simulink model "simulator_P2_2"  (R2021b)
settings: Solver=ode45  StartTime=0.0  StopTime=600  FixedStep=Ts  RelTol=1e-3  EnableMultiTasking=on
values from neighbouring files (symbols this model uses):
  A = [-0.0265 0 0.0884 0;0 -0.0265 0 0.0884; 0 0 -0.0884 0; 0 0 0 -0.0884]    [four_tanks_session2_Michal_Szabo_Michael_Brian_Damkoehler.m]
  A1 = 28    [four_tanks_session2_Michal_Szabo_Michael_Brian_Damkoehler.m]
  a1 = 0.071    [four_tanks_session2_Michal_Szabo_Michael_Brian_Damkoehler.m]
  A2 = 28    [four_tanks_session2_Michal_Szabo_Michael_Brian_Damkoehler.m]
  a2 = 0.071    [four_tanks_session2_Michal_Szabo_Michael_Brian_Damkoehler.m]
  a3 = 0.071    [four_tanks_session2_Michal_Szabo_Michael_Brian_Damkoehler.m]
  A3 = 28    [four_tanks_session2_Michal_Szabo_Michael_Brian_Damkoehler.m]
  a4 = 0.071    [four_tanks_session2_Michal_Szabo_Michael_Brian_Damkoehler.m]
  A4 = 28    [four_tanks_session2_Michal_Szabo_Michael_Brian_Damkoehler.m]
  B = [0.0833 0;0 0.0833; 0 0.0357;0.0357 0]    [four_tanks_session2_Michal_Szabo_Michael_Brian_Damkoehler.m]
  C = [1 0 0 0;0 1 0 0;0 0 1 0;0 0 0 1]    [four_tanks_session2_Michal_Szabo_Michael_Brian_Damkoehler.m]
  D = [0 0;0 0;0 0;0 0]    [four_tanks_session2_Michal_Szabo_Michael_Brian_Damkoehler.m]
  de = 0.025    [four_tanks_session2_Michal_Szabo_Michael_Brian_Damkoehler.m]
  g = 981    [four_tanks_session2_Michal_Szabo_Michael_Brian_Damkoehler.m]
  gamma1 = 0.7    [four_tanks_session2_Michal_Szabo_Michael_Brian_Damkoehler.m]
  gamma2 = 0.7    [four_tanks_session2_Michal_Szabo_Michael_Brian_Damkoehler.m]
  h10 = 4.4847    [four_tanks_session2_Michal_Szabo_Michael_Brian_Damkoehler.m]
  h20 = 4.4847    [four_tanks_session2_Michal_Szabo_Michael_Brian_Damkoehler.m]
  h30 = 0.4036    [four_tanks_session2_Michal_Szabo_Michael_Brian_Damkoehler.m]
  h40 = 0.4036    [four_tanks_session2_Michal_Szabo_Michael_Brian_Damkoehler.m]
  k1 = 3.33    [four_tanks_session2_Michal_Szabo_Michael_Brian_Damkoehler.m]
  k2 = 3.33    [four_tanks_session2_Michal_Szabo_Michael_Brian_Damkoehler.m]
  seed = [1 253 529 751]    [four_tanks_session2_Michal_Szabo_Michael_Brian_Damkoehler.m]
  Ts = 1    [four_tanks_session2_Michal_Szabo_Michael_Brian_Damkoehler.m]
  v10 = 2    [four_tanks_session2_Michal_Szabo_Michael_Brian_Damkoehler.m]
  v20 = 2    [four_tanks_session2_Michal_Szabo_Michael_Brian_Damkoehler.m]
settings Model: Creator=as  LastModifiedBy=szmis
settings SolverCC: AlgebraicLoopSolver=TrustRegion
settings DataIOCC: LimitDataPoints=on  SaveFormat=Array  SignalLoggingSaveFormat=ModelDataLogs  ReturnWorkspaceOutputs=off
settings OptimizationCC: LifeSpan=inf
settings DebuggingCC: SaveWithParameterizedLinksMsg=none  UnderspecifiedInitializationDetection=Classic  MergeDetectMultiDrivingBlocksExec=none  SolverPrmCheckMsg=warning  FcnCallInpInsideContextMsg=warning  SFUnexpectedBacktrackingDiag=warning  SFNoUnconditionalDefaultTransitionDiag=warning  SFExecutionAtInitializationDiag=none  SFMachineParentedDataDiag=warning  ArithmeticOperatorsInVariantConditions=warning
settings HardwareCC: ProdBitPerPointer=32  ProdBitPerSizeT=32  ProdBitPerPtrDiffT=32  ProdLargestAtomicFloat=None  ProdIntDivRoundTo=Undefined  ProdEndianess=Unspecified  ProdWordSize=32  ProdHWDeviceType=32-bit Generic
settings ModelReferenceCC: PropagateSignalLabelsOutOfModel=off
settings SFSimCC: SimUseLocalCustomCode=off  CustomCodeUndefinedFunction=UseInterfaceOnly
settings RTWCC: RTWUseLocalCustomCode=off
settings CodeAppCC: StateflowObjectComments=on
settings GRTTargetCC: TargetLangStandard=C89/C90 (ANSI)  CombineOutputUpdateFcns=off  GRTInterface=on
settings ConfigComp: CovMetricSettings=dw  CovSaveCumulativeToWorkspaceVar=on  CovSaveSingleToWorkspaceVar=on  CovExternalEMLEnable=off

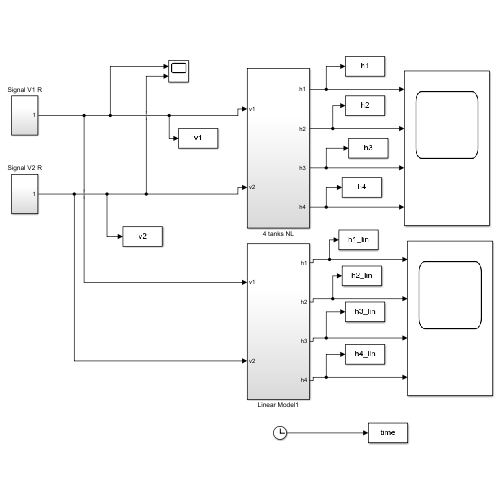
[thumbnail: Simulink's stored preview of the top-level diagram]
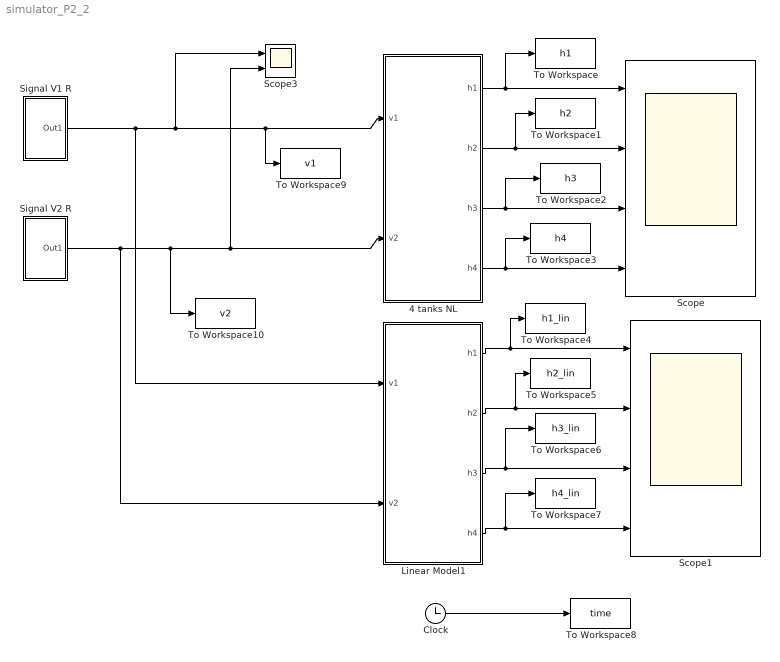
== system simulator_P2_2 ==
  4 tanks NL : Subsystem
  Clock : Clock
  Linear Model1 : Subsystem
  Scope : Scope  NumInputPorts=4
  Scope1 : Scope  NumInputPorts=4
  Scope3 : Scope  NumInputPorts=2
  Signal V1 R : Subsystem
  Signal V2 R : Subsystem
  To Workspace : ToWorkspace  VariableName=h1  SampleTime=Ts
  To Workspace1 : ToWorkspace  VariableName=h2  SampleTime=Ts
  To Workspace10 : ToWorkspace  VariableName=v2  SampleTime=Ts
  To Workspace2 : ToWorkspace  VariableName=h3  SampleTime=Ts
  To Workspace3 : ToWorkspace  VariableName=h4  SampleTime=Ts
  To Workspace4 : ToWorkspace  VariableName=h1_lin  SampleTime=Ts
  To Workspace5 : ToWorkspace  VariableName=h2_lin  SampleTime=Ts
  To Workspace6 : ToWorkspace  VariableName=h3_lin  SampleTime=Ts
  To Workspace7 : ToWorkspace  VariableName=h4_lin  SampleTime=Ts
  To Workspace8 : ToWorkspace  VariableName=time  SampleTime=Ts
  To Workspace9 : ToWorkspace  VariableName=v1  SampleTime=Ts
  wires:
  Signal V1 R/1(Out1) -> Scope3/1, 4 tanks NL/1(v1), To Workspace9/1, Linear Model1/1(v1)
  4 tanks NL/1("h1 ") -> Scope/1, To Workspace/1
  4 tanks NL/2("h2 ") -> Scope/2, To Workspace1/1
  4 tanks NL/3("h3 ") -> Scope/3, To Workspace2/1
  4 tanks NL/4("h4 ") -> Scope/4, To Workspace3/1
  Linear Model1/1(h1) -> Scope1/1, To Workspace4/1
  Linear Model1/2(h2) -> Scope1/2, To Workspace5/1
  Linear Model1/3(h3) -> Scope1/3, To Workspace6/1
  Linear Model1/4(h4) -> Scope1/4, To Workspace7/1
  Clock/1 -> To Workspace8/1
  Signal V2 R/1(Out1) -> 4 tanks NL/2(v2), Scope3/2, To Workspace10/1, Linear Model1/2(v2)

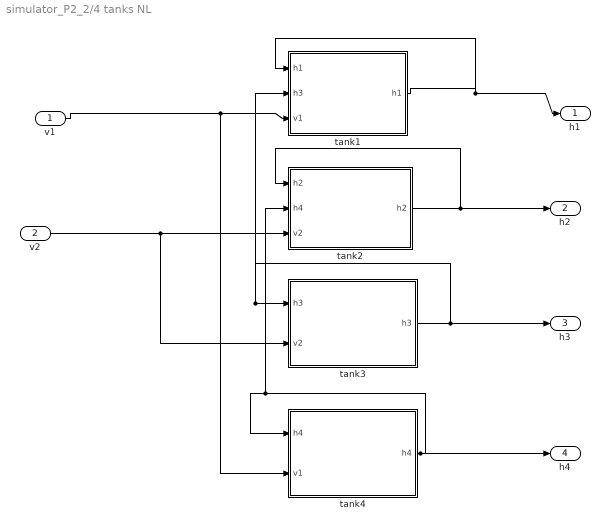
== system simulator_P2_2/4 tanks NL ==
  v1 : Inport
  v2 : Inport  Port=2
  tank1 : Subsystem
  tank2 : Subsystem
  tank3 : Subsystem
  tank4 : Subsystem
  "h1 " : Outport
  "h2 " : Outport  Port=2
  "h3 " : Outport  Port=3
  "h4 " : Outport  Port=4
  wires:
  tank4/1("h4 ") -> tank4/1(h4), tank2/2(h4), "h4 "/1
  tank3/1("h3 ") -> tank3/1(h3), tank1/2(h3), "h3 "/1
  v2/1 -> tank2/3(v2), tank3/2(v2)
  tank2/1("h2 ") -> tank2/1(h2), "h2 "/1
  v1/1 -> tank1/3(v1), tank4/2(v1)
  tank1/1("h1 ") -> tank1/1(h1), "h1 "/1

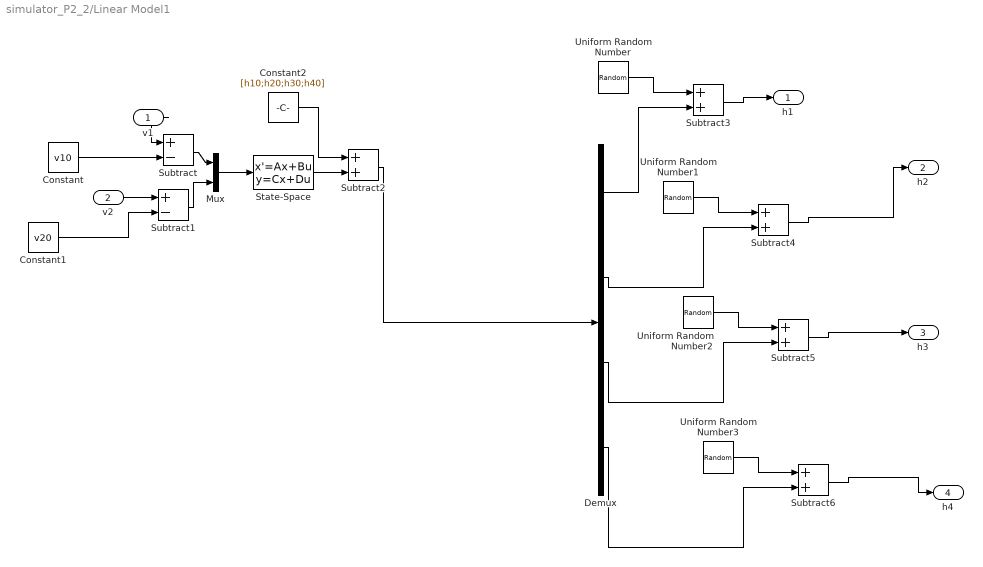
== system simulator_P2_2/Linear Model1 ==
  v1 : Inport
  v2 : Inport  Port=2
  Constant : Constant  Value=v10
  Constant1 : Constant  Value=v20
  Constant2 : Constant  Value=[h10;h20;h30;h40]
  Demux : Demux
  Mux : Mux  Inputs=2
  State-Space : StateSpace  A=A  B=B  C=C  D=D  InitialCondition=0
  Subtract : Sum  Inputs=+-
  Subtract1 : Sum  Inputs=+-
  Subtract{2..6} (5 alike) : Sum
  Uniform Random Number : UniformRandomNumber  Minimum=-de  Maximum=de  Seed=seed(1)  SampleTime=Ts
  Uniform Random Number1 : UniformRandomNumber  Minimum=-de  Maximum=de  Seed=seed(2)  SampleTime=Ts
  Uniform Random Number2 : UniformRandomNumber  Minimum=-de  Maximum=de  Seed=seed(3)  SampleTime=Ts
  Uniform Random Number3 : UniformRandomNumber  Minimum=-de  Maximum=de  Seed=seed(4)  SampleTime=Ts
  h1 : Outport
  h2 : Outport  Port=2
  h3 : Outport  Port=3
  h4 : Outport  Port=4
  wires:
  Mux/1 -> State-Space/1
  Constant/1 -> Subtract/2
  Subtract/1 -> Mux/1
  Subtract1/1 -> Mux/2
  Constant1/1 -> Subtract1/2
  Subtract2/1 -> Demux/1
  Constant2/1 -> Subtract2/1
  State-Space/1 -> Subtract2/2
  v1/1 -> Subtract/1
  v2/1 -> Subtract1/1
  Demux/1 -> Subtract3/2
  Subtract3/1 -> h1/1
  Uniform Random Number/1 -> Subtract3/1
  Demux/2 -> Subtract4/2
  Subtract4/1 -> h2/1
  Uniform Random Number1/1 -> Subtract4/1
  Demux/3 -> Subtract5/2
  Subtract5/1 -> h3/1
  Uniform Random Number2/1 -> Subtract5/1
  Demux/4 -> Subtract6/2
  Subtract6/1 -> h4/1
  Uniform Random Number3/1 -> Subtract6/1

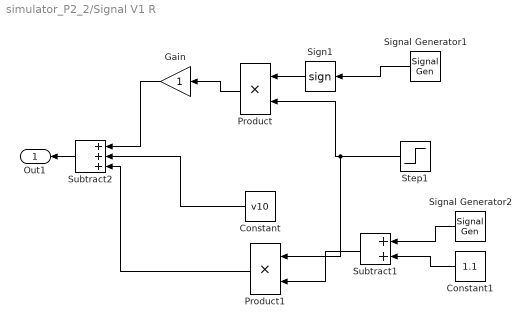
== system simulator_P2_2/Signal V1 R ==
  Constant : Constant  Value=v10
  Constant1 : Constant  Value=1.1
  Gain : Gain
  Product : Product  RndMeth=Zero
  Product1 : Product  RndMeth=Zero
  Sign1 : Signum
  Signal Generator1 : SignalGenerator  WaveForm=random  Amplitude=1.8  Frequency=200
  Signal Generator2 : SignalGenerator  WaveForm=sawtooth  Amplitude=1.1  Frequency=0.005
  Step1 : Step  Time=10  SampleTime=0
  Subtract1 : Sum
  Subtract2 : Sum  Inputs=+++
  Out1 : Outport
  wires:
  Sign1/1 -> Product/1
  Step1/1 -> Product/2, Product1/1
  Constant/1 -> Subtract2/2
  Subtract2/1 -> Out1/1
  Product/1 -> Gain/1
  Gain/1 -> Subtract2/1
  Signal Generator1/1 -> Sign1/1
  Signal Generator2/1 -> Subtract1/1
  Constant1/1 -> Subtract1/2
  Subtract1/1 -> Product1/2
  Product1/1 -> Subtract2/3

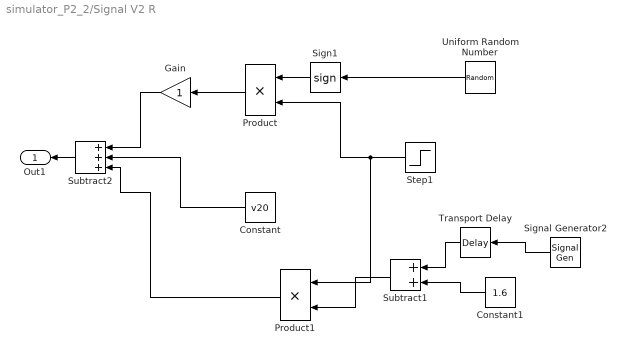
== system simulator_P2_2/Signal V2 R ==
  Constant : Constant  Value=v20
  Constant1 : Constant  Value=1.6
  Gain : Gain
  Product : Product  RndMeth=Zero
  Product1 : Product  RndMeth=Zero
  Sign1 : Signum
  Signal Generator2 : SignalGenerator  WaveForm=sawtooth  Amplitude=1.6  Frequency=0.005
  Step1 : Step  Time=10  SampleTime=0
  Subtract1 : Sum
  Subtract2 : Sum  Inputs=+++
  Transport Delay : TransportDelay  DelayTime=100
  Uniform Random Number : UniformRandomNumber  SampleTime=Ts
  Out1 : Outport
  wires:
  Uniform Random Number/1 -> Sign1/1
  Sign1/1 -> Product/1
  Step1/1 -> Product/2, Product1/1
  Constant/1 -> Subtract2/2
  Subtract2/1 -> Out1/1
  Product/1 -> Gain/1
  Gain/1 -> Subtract2/1
  Constant1/1 -> Subtract1/2
  Subtract1/1 -> Product1/2
  Product1/1 -> Subtract2/3
  Signal Generator2/1 -> Transport Delay/1
  Transport Delay/1 -> Subtract1/1

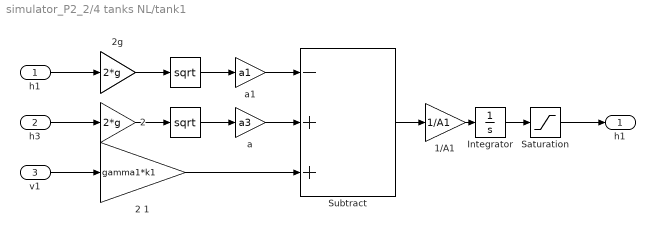
== system simulator_P2_2/4 tanks NL/tank1 ==
  h1 : Inport
  h3 : Inport  Port=2
  v1 : Inport  Port=3
  " " : Math  Operator=sqrt  SignedPower=on  SaturateOnIntegerOverflow=on
  "   " : Math  Operator=sqrt  SignedPower=on  SaturateOnIntegerOverflow=on
  1/A1 : Gain  Gain=1/A1
  "2 " : Gain  Gain=2*g
  2 1 : Gain  Gain=gamma1*k1
  2g : Gain  Gain=2*g
  Integrator : Integrator  InitialCondition=h10
  Saturation : Saturate  UpperLimit=20  LowerLimit=0
  Subtract : Sum  Inputs=-++
  a : Gain  Gain=a3
  a1 : Gain  Gain=a1
  "h1 " : Outport
  wires:
  " "/1 -> a1/1
  2g/1 -> " "/1
  a1/1 -> Subtract/1
  h1/1 -> 2g/1
  "   "/1 -> a/1
  "2 "/1 -> "   "/1
  a/1 -> Subtract/2
  h3/1 -> "2 "/1
  2 1/1 -> Subtract/3
  v1/1 -> 2 1/1
  1/A1/1 -> Integrator/1
  Saturation/1 -> "h1 "/1
  Integrator/1 -> Saturation/1
  Subtract/1 -> 1/A1/1

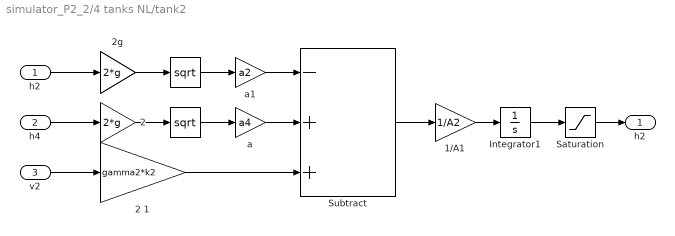
== system simulator_P2_2/4 tanks NL/tank2 ==
  h2 : Inport
  h4 : Inport  Port=2
  v2 : Inport  Port=3
  " " : Math  Operator=sqrt  SignedPower=on  SaturateOnIntegerOverflow=on
  "   " : Math  Operator=sqrt  SignedPower=on  SaturateOnIntegerOverflow=on
  1/A1 : Gain  Gain=1/A2
  "2 " : Gain  Gain=2*g
  2 1 : Gain  Gain=gamma2*k2
  2g : Gain  Gain=2*g
  Integrator1 : Integrator  InitialCondition=h20
  Saturation : Saturate  UpperLimit=20  LowerLimit=0
  Subtract : Sum  Inputs=-++
  a : Gain  Gain=a4
  a1 : Gain  Gain=a2
  "h2 " : Outport
  wires:
  1/A1/1 -> Integrator1/1
  v2/1 -> 2 1/1
  2 1/1 -> Subtract/3
  h4/1 -> "2 "/1
  a/1 -> Subtract/2
  "2 "/1 -> "   "/1
  "   "/1 -> a/1
  h2/1 -> 2g/1
  a1/1 -> Subtract/1
  2g/1 -> " "/1
  " "/1 -> a1/1
  Saturation/1 -> "h2 "/1
  Integrator1/1 -> Saturation/1
  Subtract/1 -> 1/A1/1

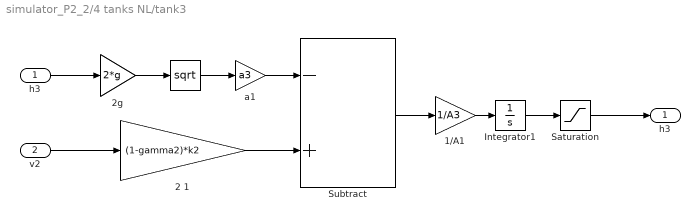
== system simulator_P2_2/4 tanks NL/tank3 ==
  h3 : Inport
  v2 : Inport  Port=2
  " " : Math  Operator=sqrt  SignedPower=on  SaturateOnIntegerOverflow=on
  1/A1 : Gain  Gain=1/A3
  2 1 : Gain  Gain=(1-gamma2)*k2
  2g : Gain  Gain=2*g
  Integrator1 : Integrator  InitialCondition=h30
  Saturation : Saturate  UpperLimit=20  LowerLimit=0
  Subtract : Sum  Inputs=-+
  a1 : Gain  Gain=a3
  "h3 " : Outport
  wires:
  " "/1 -> a1/1
  2g/1 -> " "/1
  a1/1 -> Subtract/1
  h3/1 -> 2g/1
  2 1/1 -> Subtract/2
  v2/1 -> 2 1/1
  1/A1/1 -> Integrator1/1
  Saturation/1 -> "h3 "/1
  Subtract/1 -> 1/A1/1
  Integrator1/1 -> Saturation/1

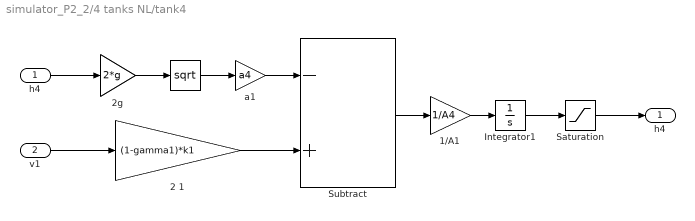
== system simulator_P2_2/4 tanks NL/tank4 ==
  h4 : Inport
  v1 : Inport  Port=2
  " " : Math  Operator=sqrt  SignedPower=on  SaturateOnIntegerOverflow=on
  1/A1 : Gain  Gain=1/A4
  2 1 : Gain  Gain=(1-gamma1)*k1
  2g : Gain  Gain=2*g
  Integrator1 : Integrator  InitialCondition=h40
  Saturation : Saturate  UpperLimit=20  LowerLimit=0
  Subtract : Sum  Inputs=-+
  a1 : Gain  Gain=a4
  "h4 " : Outport
  wires:
  1/A1/1 -> Integrator1/1
  v1/1 -> 2 1/1
  2 1/1 -> Subtract/2
  h4/1 -> 2g/1
  a1/1 -> Subtract/1
  2g/1 -> " "/1
  " "/1 -> a1/1
  Saturation/1 -> "h4 "/1
  Subtract/1 -> 1/A1/1
  Integrator1/1 -> Saturation/1
